simulink model "diff_drive_sim"  (Simulink 8.7)
settings: Solver=VariableStepAuto  SolverMode=SingleTasking  StartTime=0.0  StopTime=489.5  RelTol=1e-3
values from neighbouring files (symbols this model uses):
  a = 4    [bicycle.m]    (also in diff_drive.m)
  d = 0.01    [bicycle.m]    (also in diff_drive.m = 0.075)
  K_theta = 1    [bicycle.m]    (also in diff_drive.m = 0.001)
  Kp = 7    [bicycle.m]    (also in diff_drive.m = 1)
  Kx = 30    [bicycle.m]    (also in diff_drive.m = 15)
  Ky = 30    [bicycle.m]    (also in diff_drive.m = 150)
  theta0 = pi/2    (= 1.57079632679)    [bicycle.m]    (also in diff_drive.m)
  w = 0.1    [bicycle.m]    (also in diff_drive.m)
  x0 = a    (= 4)    [bicycle.m]    (also in diff_drive.m)
  y0 = 0    [bicycle.m]    (also in diff_drive.m)
settings Model: Creator=olivier  LastModifiedBy=sanjy
settings SolverCC: ZeroCrossAlgorithm=Adaptive
settings DataIOCC: LimitDataPoints=off
settings DebuggingCC: UnderspecifiedInitializationDetection=Simplified  MergeDetectMultiDrivingBlocksExec=error  MaskedZcDiagnostic=none  SFUnexpectedBacktrackingDiag=error  SFNoUnconditionalDefaultTransitionDiag=error
settings HardwareCC: ProdBitPerPointer=64  ProdLargestAtomicFloat=Float  ProdIntDivRoundTo=Zero  ProdEndianess=LittleEndian  ProdWordSize=64  ProdHWDeviceType=Intel->x86-64 (Windows64)
settings ModelReferenceCC: PropagateSignalLabelsOutOfModel=on
settings SFSimCC: SimUseLocalCustomCode=on
settings RTWCC: RTWUseLocalCustomCode=on
settings GRTTargetCC: TargetLangStandard=C99 (ISO)  GeneratePreprocessorConditionals=Use local settings
settings ConfigComp: CovMetricSettings=dwe  CovHtmlReporting=off  CovSaveCumulativeToWorkspaceVar=off  CovSaveSingleToWorkspaceVar=off  CovModelRefEnable=off  CovExternalEMLEnable=on

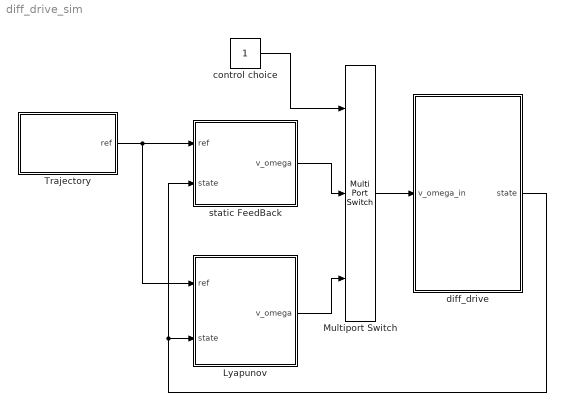
== system diff_drive_sim ==
  Lyapunov : Subsystem
  Multiport Switch : MultiPortSwitch  Inputs=2
  Trajectory : Subsystem  TreatAsAtomicUnit=on
  control choice : Constant
  diff_drive : Subsystem  mask{base=0.5, base_error=0, radius=0.2, radius_error=0, omega_max=127}
      mask prompts: base_error "Base error in percent"; radius_error "Radius error in percent"; omega_max "Wheel Max Velocity"
  static FeedBack : Subsystem
  wires:
  Trajectory/1(ref) -> Lyapunov/1(ref), static FeedBack/1(ref)
  static FeedBack/1(v_omega) -> Multiport Switch/2
  Multiport Switch/1 -> diff_drive/1(v_omega_in)
  control choice/1 -> Multiport Switch/1
  diff_drive/1(state) -> Lyapunov/2(state), static FeedBack/2(state)
  Lyapunov/1(v_omega) -> Multiport Switch/3

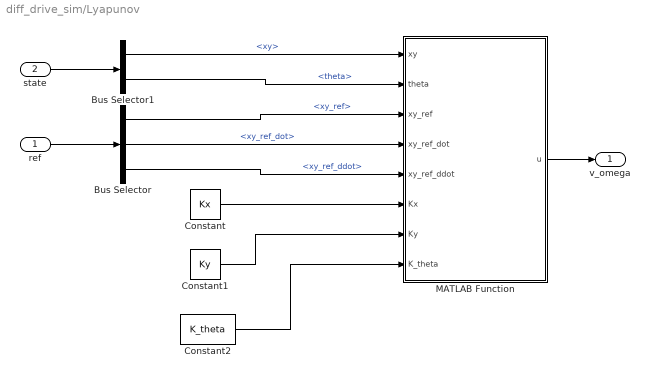
== system diff_drive_sim/Lyapunov ==
  ref : Inport
  state : Inport  Port=2
  Bus Selector : BusSelector  OutputSignals=xy_ref,xy_ref_dot,xy_ref_ddot
  Bus Selector1 : BusSelector  OutputSignals=xy,theta
  Constant : Constant  Value=Kx
  Constant1 : Constant  Value=Ky
  Constant2 : Constant  Value=K_theta
  MATLAB Function : MATLAB Function  TreatAsAtomicUnit=on
  v_omega : Outport
  wires:
  MATLAB Function/1(u) -> v_omega/1
  ref/1 -> Bus Selector/1
  state/1 -> Bus Selector1/1
  Bus Selector/2 -> MATLAB Function/4(xy_ref_dot)  "<xy_ref_dot>"
  Bus Selector/1 -> MATLAB Function/3(xy_ref)  "<xy_ref>"
  Bus Selector/3 -> MATLAB Function/5(xy_ref_ddot)  "<xy_ref_ddot>"
  Bus Selector1/1 -> MATLAB Function/1(xy)  "<xy>"
  Bus Selector1/2 -> MATLAB Function/2(theta)  "<theta>"
  Constant2/1 -> MATLAB Function/8(K_theta)
  Constant1/1 -> MATLAB Function/7(Ky)
  Constant/1 -> MATLAB Function/6(Kx)

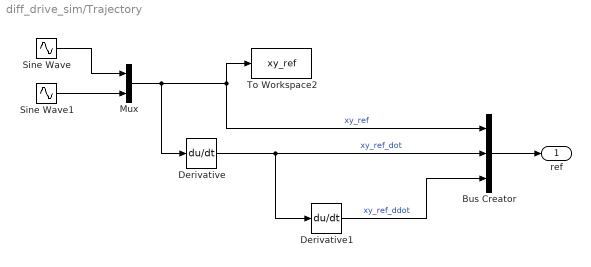
== system diff_drive_sim/Trajectory ==
  Bus Creator : BusCreator  Inputs=3
  Derivative : Derivative
  Derivative1 : Derivative
  Mux : Mux  Inputs=2
  Sine Wave : Sin  Amplitude=a  Frequency=w  Phase=pi/2  SampleTime=0
  Sine Wave1 : Sin  Amplitude=a  Frequency=w  SampleTime=0
  To Workspace2 : ToWorkspace  VariableName=xy_ref  SampleTime=-1
      settings: Save2DSignal=2-D array (concatenate along first dimension)
  ref : Outport
  wires:
  Bus Creator/1 -> ref/1
  Mux/1 -> Derivative/1, Bus Creator/1, To Workspace2/1  "xy_ref"
  Derivative/1 -> Bus Creator/2, Derivative1/1  "xy_ref_dot"
  Derivative1/1 -> Bus Creator/3  "xy_ref_ddot"
  Sine Wave/1 -> Mux/1
  Sine Wave1/1 -> Mux/2

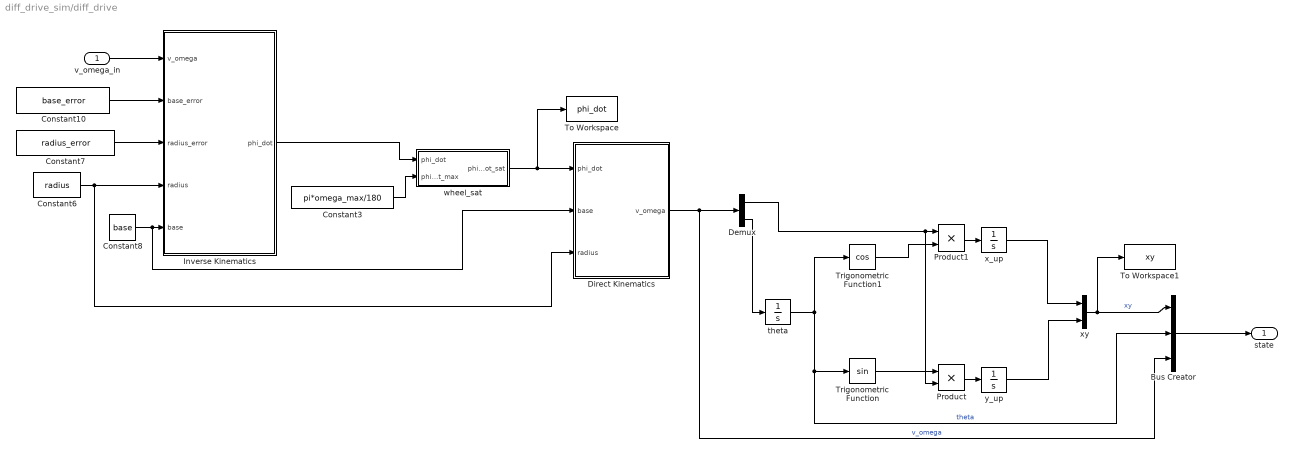
== system diff_drive_sim/diff_drive ==
  v_omega_in : Inport
  Bus Creator : BusCreator  Inputs=3
  Constant10 : Constant  Value=base_error
  Constant3 : Constant  Value=pi*omega_max/180
  Constant6 : Constant  Value=radius
  Constant7 : Constant  Value=radius_error
  Constant8 : Constant  Value=base
  Demux : Demux  Outputs=2
  Direct Kinematics : MATLAB Function  TreatAsAtomicUnit=on
  Inverse Kinematics : MATLAB Function  TreatAsAtomicUnit=on
  Product : Product
  Product1 : Product
  To Workspace : ToWorkspace  VariableName=phi_dot  SampleTime=-1
      settings: Save2DSignal=2-D array (concatenate along first dimension)
  To Workspace1 : ToWorkspace  VariableName=xy  SampleTime=-1
      settings: Save2DSignal=2-D array (concatenate along first dimension)
  Trigonometric Function : Trigonometry
  Trigonometric Function1 : Trigonometry  Operator=cos
  theta : Integrator  InitialCondition=theta0
  wheel_sat : Subsystem
  x_up : Integrator  InitialCondition=x0
  xy : Mux  Inputs=2
  y_up : Integrator  InitialCondition=y0
  state : Outport
  wires:
  theta/1 -> Trigonometric Function1/1, Trigonometric Function/1, Bus Creator/2  "theta"
  Trigonometric Function1/1 -> Product1/2
  Trigonometric Function/1 -> Product/1
  Product/1 -> y_up/1
  Product1/1 -> x_up/1
  x_up/1 -> xy/1
  Constant3/1 -> wheel_sat/2(phi_dot_max)
  Direct Kinematics/1(v_omega) -> Bus Creator/3, Demux/1  "v_omega"
  Demux/1 -> Product/2, Product1/1
  Demux/2 -> theta/1
  y_up/1 -> xy/2
  wheel_sat/1(phi_dot_sat) -> Direct Kinematics/1(phi_dot), To Workspace/1
  xy/1 -> Bus Creator/1, To Workspace1/1  "xy"
  Bus Creator/1 -> state/1
  Inverse Kinematics/1(phi_dot) -> wheel_sat/1(phi_dot)
  v_omega_in/1 -> Inverse Kinematics/1(v_omega)
  Constant10/1 -> Inverse Kinematics/2(base_error)
  Constant7/1 -> Inverse Kinematics/3(radius_error)
  Constant6/1 -> Inverse Kinematics/4(radius), Direct Kinematics/3(radius)
  Constant8/1 -> Direct Kinematics/2(base), Inverse Kinematics/5(base)

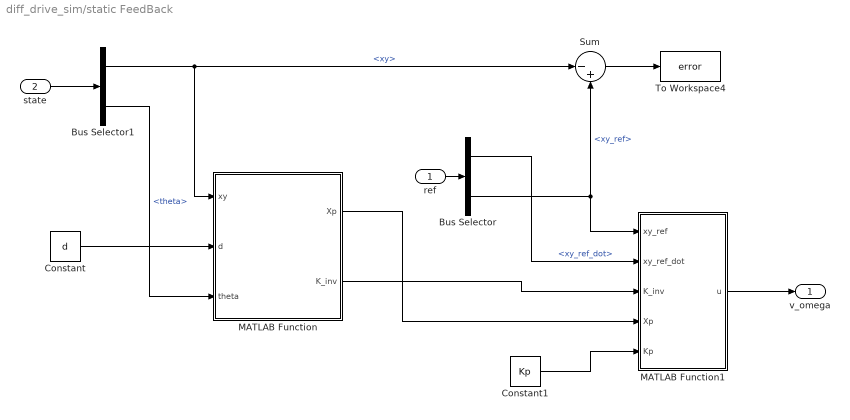
== system diff_drive_sim/static FeedBack ==
  ref : Inport
  state : Inport  Port=2
  Bus Selector : BusSelector  OutputSignals=xy_ref_dot,xy_ref
  Bus Selector1 : BusSelector  OutputSignals=xy,theta
  Constant : Constant  Value=d
  Constant1 : Constant  Value=Kp
  MATLAB Function : MATLAB Function  TreatAsAtomicUnit=on
  MATLAB Function1 : MATLAB Function  TreatAsAtomicUnit=on
  Sum : Sum  Inputs=|-+
  To Workspace4 : ToWorkspace  VariableName=error  SampleTime=-1
      settings: Save2DSignal=2-D array (concatenate along first dimension)
  v_omega : Outport
  wires:
  ref/1 -> Bus Selector/1
  state/1 -> Bus Selector1/1
  Bus Selector/2 -> MATLAB Function1/1(xy_ref), Sum/2  "<xy_ref>"
  Bus Selector1/1 -> MATLAB Function/1(xy), Sum/1  "<xy>"
  Sum/1 -> To Workspace4/1
  MATLAB Function1/1(u) -> v_omega/1
  Bus Selector1/2 -> MATLAB Function/3(theta)  "<theta>"
  Constant1/1 -> MATLAB Function1/5(Kp)
  MATLAB Function/1(Xp) -> MATLAB Function1/4(Xp)
  MATLAB Function/2(K_inv) -> MATLAB Function1/3(K_inv)
  Bus Selector/1 -> MATLAB Function1/2(xy_ref_dot)  "<xy_ref_dot>"
  Constant/1 -> MATLAB Function/2(d)

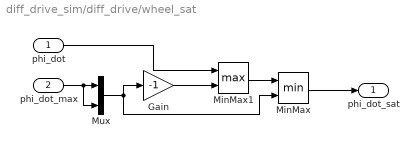
== system diff_drive_sim/diff_drive/wheel_sat ==
  phi_dot : Inport
  phi_dot_max : Inport  Port=2
  Gain : Gain  Gain=-1
  MinMax : MinMax  Inputs=2
  MinMax1 : MinMax  Function=max  Inputs=2
  Mux : Mux  Inputs=2
  phi_dot_sat : Outport
  wires:
  Gain/1 -> MinMax1/2
  MinMax/1 -> phi_dot_sat/1
  phi_dot_max/1 -> Mux/2, Mux/1
  phi_dot/1 -> MinMax1/1
  MinMax1/1 -> MinMax/1
  Mux/1 -> MinMax/2, Gain/1

== matlab function diff_drive/Inverse Kinematics ==
  data: v_omega input double; base_error input double; radius_error input double; radius input double; phi_dot output double; base input double
function phi_dot = ik(v_omega, base_error, radius_error, radius, base)

base = base * (1+base_error*0.01);
radius = radius * (1+radius_error*0.01);

phi_dot = [(v_omega(1)+base*v_omega(2))/radius; (v_omega(1)-base*v_omega(2))/radius];

== matlab function static FeedBack/MATLAB Function ==
  data: xy input double; d input double; theta input double; Xp output double; K_inv output double
function [Xp,K_inv] = fcn(xy,d,theta)

xp= xy(1) + d*cos(theta);
yp= xy(2) + d*sin(theta);
Xp=[xp;yp];

% k_inv calculation
K = [cos(theta), -d * sin(theta); sin(theta),d * cos(theta)];
K_inv= inv(K);

== matlab function static FeedBack/MATLAB Function1 ==
  data: xy_ref input double; u output double; xy_ref_dot input double; K_inv input double; Xp input double; Kp input double
function u = fcn(xy_ref,xy_ref_dot,K_inv,Xp,Kp)

error = xy_ref - Xp;

xp_star = xy_ref_dot + (Kp*error);

u = K_inv*xp_star ;

== matlab function diff_drive/Direct Kinematics ==
  data: phi_dot input double; v_omega output double; base input double; radius input double
function v_omega = dk(phi_dot, base, radius)

v_omega = [radius*(phi_dot(1)+phi_dot(2))/2; radius*(phi_dot(1)-phi_dot(2))/(2*base)];

== matlab function Lyapunov/MATLAB Function ==
  data: xy input double; u output double; theta input double; xy_ref input double; xy_ref_dot input double; xy_ref_ddot input double; Kx input double; Ky input double; K_theta input double
function u = fcn(xy,theta,xy_ref,xy_ref_dot,xy_ref_ddot,Kx,Ky,K_theta)

xe = cos(theta)*(xy_ref(1)-xy(1)) + sin(theta)*(xy_ref(2)-xy(2));

ye = -sin(theta)*(xy_ref(1)-xy(1)) + cos(theta)*(xy_ref(2)-xy(end));

theta_e = atan2(xy_ref_dot(2),xy_ref_dot(1)) - theta;

% if (-pi<theta_e)
%     
%     theta_e = theta_e + pi;
%     
% elseif(theta_e>pi)
%     
%     theta_e = theta_e - pi;
%     
% end 

theta_e = theta_e -2*pi*floor((theta_e+pi)/(2*pi));

vr = (xy_ref_dot(1)*cos(theta)) + (xy_ref_dot(2)*sin(theta));

if vr == 0
    
    wr = 0;
    
else
    
wr = (xy_ref_dot(1)*xy_ref_ddot(2) - xy_ref_ddot(1)*xy_ref_dot(2))/vr^2;

end

v = vr*cos(theta_e) + Kx*xe;

w = wr + (Ky*ye*vr*sin(theta_e)/theta_e) + (K_theta*theta_e);

u = [v;w];
